simulink model "SimiSnake3"  (R2018b)
settings: Solver=VariableStepAuto  StartTime=0.0  StopTime=10.0  RelTol=1e-3  EnableMultiTasking=on
PreLoadFcn:
  | robotParameters;
undefined symbols (not defined in the file or in its folder): X, Y, Z
libraries: sm_lib x38, nesl_utility x25, simulink x6
settings Model: Creator=Jake  LastModifiedBy=Jake
settings DataIOCC: LimitDataPoints=on
settings OptimizationCC: LifeSpan=inf
settings DebuggingCC: AllowSymbolicDim=off  SFUnexpectedBacktrackingDiag=warning  SFNoUnconditionalDefaultTransitionDiag=warning  SFExecutionAtInitializationDiag=none
settings SFSimCC: SimUseLocalCustomCode=off
settings RTWCC: RTWUseLocalCustomCode=off
settings CodeAppCC: StateflowObjectComments=on
settings GRTTargetCC: TargetLangStandard=C89/C90 (ANSI)  GeneratePreprocessorConditionals=Disable all
settings ConfigComp: CovMetricSettings=dw  CovHtmlReporting=on  CovSaveCumulativeToWorkspaceVar=on  CovSaveSingleToWorkspaceVar=on  CovExternalEMLEnable=off  CovSFcnEnable=off
settings SimscapeCC: SimscapeNominalValues="[{\"value\":\"10\",\"unit\":\"V\"},{\"value\":\"1\",\"unit\":\"A\"},{\"value\":\"10\",\"unit\":\"N*m\"},{\"value\":\"10\",\"unit\":\"bar\"},{\"value\":\"100\",\"unit\":\"kJ/kg\"},{\"value\":\"1\",\"unit\":\"kW\"},{\"value\":\"300\",\"unit\":\"K\"},{\"value\":\"100\",\"unit\":\"cm^3/s\"},{\"value\":\"1\",\"unit\":\"kN\"},{\"value\":\"1\",\"unit\":\"g/cm^3\"},{\"value\":\"1\",\"unit\":\"l\"},{\"value\":\"1\",\"unit\":\"cm^2\"},{\"value\":\"60\",\"unit\":\"Hz\"}]"  SimscapeLogType=all  SimscapeLogDataHistory=10000
settings ConfigurationSet: Description=SimMechanics 2G

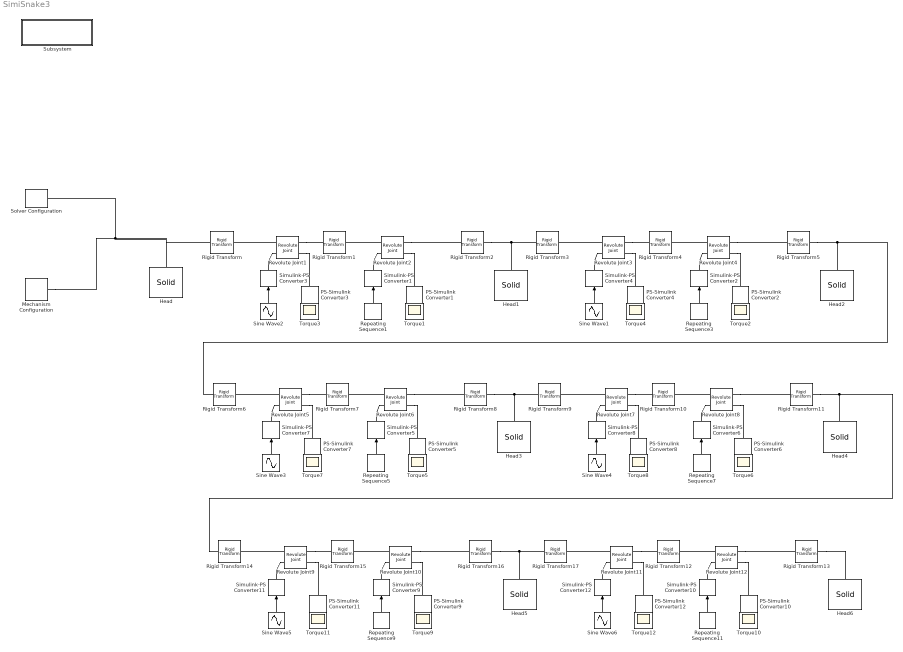
== system SimiSnake3 ==
  Head : sm_lib/Body Elements/Solid  InertiaType=CalculateFromGeometry  Mass=1  MassUnits=kg  CenterOfMass=[0 0 0]  CenterOfMassUnits=m  MomentsOfInertia=[1 1 1]  MomentsOfInertiaUnits=kg*m^2  ProductsOfInertia=[0 0 0]  ProductsOfInertiaUnits=kg*m^2  BasedOnType=Density  Density=0  DensityUnits=kg/m^3  DoExposeReferenceFrame=on  SerializedFrames=<Frames/>  GraphicType=FromGeometry  MarkerShape=Sphere  MarkerSize=10  GraphicVisPropType=SimpleVisualProperties  GraphicDiffuseColor=[1.0 0.0 0.2]  GraphicSpecularColor=[0.5 0.5 0.5 1.0]  GraphicAmbientColor=[0.15 0.15 0.15 1.0]  GraphicEmissiveColor=[0.0 0.0 0.0 1.0]  GraphicShininess=75  GraphicOpacity=1.0  GeometryShape=Cylinder  RectangleSize=[1 1]  RectangleSizeUnits=m  BrickDimensions=[1 1 1]  BrickDimensionUnits=m  CylinderRadius=1  CylinderRadiusUnits=cm  CylinderLength=10  CylinderLengthUnits=cm  SphereRadius=1  SphereRadiusUnits=m  EllipsoidRadii=[1 1 1]  EllipsoidRadiiUnits=m  ExtrusionCrossSection=[1 1; -1 1; -1 -1; 1 -1]  ExtrusionCrossSectionUnits=m  ExtrusionLength=1  ExtrusionLengthUnits=m  PolygonNumSides=3  PolygonOuterRadius=1  PolygonOuterRadiusUnits=m  ExtGeomFileType=STEP  ExtGeomFileUnits=m  RevolutionCrossSection=[1 1; 1 -1; 2 -1; 2 1]  RevolutionCrossSectionUnits=m  RevolutionExtent=Full  RevolutionAngle=180  RevolutionAngleUnits=deg
  Head{1..6} (6 alike) : sm_lib/Body Elements/Solid  InertiaType=CalculateFromGeometry  Mass=1  MassUnits=kg  CenterOfMass=[0 0 0]  CenterOfMassUnits=m  MomentsOfInertia=[1 1 1]  MomentsOfInertiaUnits=kg*m^2  ProductsOfInertia=[0 0 0]  ProductsOfInertiaUnits=kg*m^2  BasedOnType=Density  Density=500  DensityUnits=kg/m^3  DoExposeReferenceFrame=on  SerializedFrames=<Frames/>  GraphicType=FromGeometry  MarkerShape=Sphere  MarkerSize=10  GraphicVisPropType=SimpleVisualProperties  GraphicDiffuseColor=[1.0 1.0 0.2]  GraphicSpecularColor=[0.5 0.5 0.5 1.0]  GraphicAmbientColor=[0.15 0.15 0.15 1.0]  GraphicEmissiveColor=[0.0 0.0 0.0 1.0]  GraphicShininess=75  GraphicOpacity=1.0  GeometryShape=Cylinder  RectangleSize=[1 1]  RectangleSizeUnits=m  BrickDimensions=[1 1 1]  BrickDimensionUnits=m  CylinderRadius=1  CylinderRadiusUnits=cm  CylinderLength=10  CylinderLengthUnits=cm  SphereRadius=1  SphereRadiusUnits=m  EllipsoidRadii=[1 1 1]  EllipsoidRadiiUnits=m  ExtrusionCrossSection=[1 1; -1 1; -1 -1; 1 -1]  ExtrusionCrossSectionUnits=m  ExtrusionLength=1  ExtrusionLengthUnits=m  PolygonNumSides=3  PolygonOuterRadius=1  PolygonOuterRadiusUnits=m  ExtGeomFileType=STEP  ExtGeomFileUnits=m  RevolutionCrossSection=[1 1; 1 -1; 2 -1; 2 1]  RevolutionCrossSectionUnits=m  RevolutionExtent=Full  RevolutionAngle=180  RevolutionAngleUnits=deg
  Mechanism Configuration : sm_lib/Utilities/Mechanism Configuration  UniformGravity=Constant  GravityVector=[0 0 0]  GravityUnits=m/s^2  LinearizationDelta=0.001
  PS-Simulink Converter{1..12} (12 alike) : nesl_utility/PS-Simulink Converter  PhysicalDomain=network_engine_domain  SubClassName=ps_output  LeftPortType=input  RightPortType=output  PseudoPeriodic=off  Frequencies=[]  Unit=N*m  AffineConversion=off
  Repeating Sequence1 : simulink/Sources/Repeating Sequence  rep_seq_t=[0 1 2 3 4 5 6 7 8 9 10]  rep_seq_y=[0 -0 -20 -0 20 -0 -20 -0 20 -0 -20]
  Repeating Sequence{3,5,7,9,11} (5 alike) : simulink/Sources/Repeating Sequence  rep_seq_t=[0 1 2 3 4 5 6 7 8 9 10]  rep_seq_y=[0 -0 0 -0 0 -0 0 -0 0 -0 0]
  Revolute Joint{1..12} (12 alike) : sm_lib/Joints/Revolute Joint  SenseConstraintForce=off  SenseConstraintForceX=off  SenseConstraintForceY=off  SenseConstraintForceZ=off  SenseConstraintTorque=off  SenseConstraintTorqueX=off  SenseConstraintTorqueY=off  SenseConstraintTorqueZ=off  SenseTotalForce=off  SenseTotalForceX=off  SenseTotalForceY=off  SenseTotalForceZ=off  SenseTotalTorque=off  SenseTotalTorqueX=off  SenseTotalTorqueY=off  SenseTotalTorqueZ=off  CompositeWrenchDir=FollowerOnBase  CompositeWrenchFrame=BaseFrame  EquilibriumPosition=0  EquilibriumPositionUnits=deg  SpringStiffness=0  SpringStiffnessUnits=N*m/deg  DampingCoefficient=0  DampingCoefficientUnits=N*m/(deg/s)  TorqueActuationMode=ComputedTorque  MotionActuationMode=InputMotion  SensePosition=off  SenseVelocity=off  SenseAcceleration=off  SenseTorqueForce=on  PositionTargetSpecify=off  PositionTargetPriority=High  PositionTargetValue=30  PositionTargetValueUnits=deg  VelocityTargetSpecify=off  VelocityTargetPriority=High  VelocityTargetValue=0  VelocityTargetValueUnits=deg/s
  Rigid Transform{,3,6,9,14,17} (6 alike) : sm_lib/Frames and Transforms/Rigid Transform  TranslationMethod=StandardAxis  TranslationStandardOffset=5  TranslationLengthUnit=cm  TranslationStandardAxis=-Z  TranslationCartesianOffset=[0 0 0]  TranslationROffset=0  TranslationROffsetUnits=m  TranslationZOffset=0  TranslationZOffsetUnits=m  TranslationThetaOffset=0  TranslationThetaOffsetUnits=deg  RotationMethod=StandardAxis  RotationAngleUnits=deg  RotationStandardAxis=+X  RotationAngle=90  RotationArbitraryAxis=[0 0 1]  FollAlignAxisA=+X  BaseAlignAxisA=+Y  FollAlignAxisB=+Y  BaseAlignAxisB=+Z  RotationSequenceAxes=FollowerAxes  RotationSequence=XYX  RotationSequenceAngles=[0 0 0]  RotationSequenceAnglesUnits=deg  RotationMatrix=[1 0 0; 0 1 0; 0 0 1]
  Rigid Transform{1,4,7,10,12,15} (6 alike) : sm_lib/Frames and Transforms/Rigid Transform  TranslationMethod=None  TranslationStandardOffset=5  TranslationLengthUnit=cm  TranslationStandardAxis=-Z  TranslationCartesianOffset=[0 0 0]  TranslationROffset=0  TranslationROffsetUnits=m  TranslationZOffset=0  TranslationZOffsetUnits=m  TranslationThetaOffset=0  TranslationThetaOffsetUnits=deg  RotationMethod=StandardAxis  RotationAngleUnits=deg  RotationStandardAxis=+X  RotationAngle=90  RotationArbitraryAxis=[0 0 1]  FollAlignAxisA=+X  BaseAlignAxisA=+Y  FollAlignAxisB=+Y  BaseAlignAxisB=+Z  RotationSequenceAxes=FollowerAxes  RotationSequence=XYX  RotationSequenceAngles=[0 0 0]  RotationSequenceAnglesUnits=deg  RotationMatrix=[1 0 0; 0 1 0; 0 0 1]
  Rigid Transform{2,5,8,11,13,16} (6 alike) : sm_lib/Frames and Transforms/Rigid Transform  TranslationMethod=StandardAxis  TranslationStandardOffset=5  TranslationLengthUnit=cm  TranslationStandardAxis=+Z  TranslationCartesianOffset=[0 0 0]  TranslationROffset=0  TranslationROffsetUnits=m  TranslationZOffset=0  TranslationZOffsetUnits=m  TranslationThetaOffset=0  TranslationThetaOffsetUnits=deg  RotationMethod=StandardAxis  RotationAngleUnits=deg  RotationStandardAxis=-X  RotationAngle=180  RotationArbitraryAxis=[0 0 1]  FollAlignAxisA=+X  BaseAlignAxisA=+Y  FollAlignAxisB=+Y  BaseAlignAxisB=+Z  RotationSequenceAxes=FollowerAxes  RotationSequence=XYX  RotationSequenceAngles=[0 0 0]  RotationSequenceAnglesUnits=deg  RotationMatrix=[1 0 0; 0 1 0; 0 0 1]
  Simulink-PS Converter{1..12} (12 alike) : nesl_utility/Simulink-PS Converter  PhysicalDomain=network_engine_domain  SubClassName=ps_input  LeftPortType=input  RightPortType=output  PseudoPeriodic=off  Frequencies=[]  NoiseDistribution=none  NoiseParameters=[]  Unit=deg  AffineConversion=off  FilteringAndDerivatives=filter  SimscapeFilterOrder=2  InputFilterTimeConstant=.01  UdotUserProvided=1
  Sine Wave1 : Sin  Amplitude=80  Frequency=5  Phase=-pi/2  SampleTime=0
  Sine Wave2 : Sin  Amplitude=80  Frequency=5  SampleTime=0
  Sine Wave3 : Sin  Amplitude=80  Frequency=5  Phase=-pi*(2/2)  SampleTime=0
  Sine Wave4 : Sin  Amplitude=80  Frequency=5  Phase=-pi*(3/2)  SampleTime=0
  Sine Wave5 : Sin  Amplitude=80  Frequency=5  Phase=-pi*(4/2)  SampleTime=0
  Sine Wave6 : Sin  Amplitude=80  Frequency=5  Phase=-pi*(5/2)  SampleTime=0
  Solver Configuration : nesl_utility/Solver Configuration  PhysicalDomain=network_engine_domain  SubClassName=solver  LeftPortType=input  RightPortType=generic  Tones=[]  Harmonics=[]  SimulateNoise=off  Profile=off  UseLocalSampling=off  EnableSwitchedLinearOptims=on  FrequencyDomain=off  UseCCode=off  RelTol=0.001  AbsTol=1e-06  MinStep=1e-09  ToWorkspace=off  RevertToSquareIcSolve=off  NumHomotopyIterations=100  PhasorMode=off  PhasorModeNumHarmonics=1  DoDC=off  ResidualTolerance=1e-09  UseLocalSolver=off  LocalSolverChoice=NE_BACKWARD_EULER_ADVANCER  LocalSolverSampleTime=0.001  DoFixedCost=off  MaxNonlinIter=3  MaxModeIter=2  LinearAlgebra=Sparse  EquationFormulation=NE_TIME_EF  DelaysMemoryBudget=1024  AutomaticFiltering=on  FilteringTimeConstant=0.001  PartitionStorageMethod=AS_NEEDED  PartitionMemoryBudget=1024
  Subsystem : Subsystem
      settings: OpenFcn=open_system('sm_lib')
      mask Display: disp(sprintf('Open Simscape Multibody\nLibrary'));
  Torque{1..12} (12 alike) : Scope
  wires:
  Sine Wave2/1 -> Simulink-PS Converter3/1
  PS-Simulink Converter3/1 -> Torque3/1
  Repeating Sequence1/1 -> Simulink-PS Converter1/1
  PS-Simulink Converter1/1 -> Torque1/1
  Repeating Sequence3/1 -> Simulink-PS Converter2/1
  PS-Simulink Converter2/1 -> Torque2/1
  Sine Wave1/1 -> Simulink-PS Converter4/1
  PS-Simulink Converter4/1 -> Torque4/1
  Repeating Sequence5/1 -> Simulink-PS Converter5/1
  PS-Simulink Converter5/1 -> Torque5/1
  Sine Wave4/1 -> Simulink-PS Converter8/1
  PS-Simulink Converter6/1 -> Torque6/1
  Repeating Sequence7/1 -> Simulink-PS Converter6/1
  PS-Simulink Converter8/1 -> Torque8/1
  Sine Wave3/1 -> Simulink-PS Converter7/1
  PS-Simulink Converter7/1 -> Torque7/1
  PS-Simulink Converter9/1 -> Torque9/1
  Repeating Sequence9/1 -> Simulink-PS Converter9/1
  Sine Wave6/1 -> Simulink-PS Converter12/1
  Sine Wave5/1 -> Simulink-PS Converter11/1
  PS-Simulink Converter11/1 -> Torque11/1
  Repeating Sequence11/1 -> Simulink-PS Converter10/1
  PS-Simulink Converter12/1 -> Torque12/1
  PS-Simulink Converter10/1 -> Torque10/1
  connections:
  Mechanism Configuration/RConn1 -- Rigid Transform/LConn1 -- Head/RConn1 -- Solver Configuration/RConn1
  Revolute Joint1/RConn2 -- PS-Simulink Converter3/LConn1
  Simulink-PS Converter3/RConn1 -- Revolute Joint1/LConn2
  Revolute Joint1/RConn1 -- Rigid Transform1/LConn1
  Revolute Joint1/LConn1 -- Rigid Transform/RConn1
  Rigid Transform2/RConn1 -- Rigid Transform3/LConn1 -- Head1/RConn1
  Revolute Joint2/LConn1 -- Rigid Transform1/RConn1
  Revolute Joint2/RConn1 -- Rigid Transform2/LConn1
  Revolute Joint2/RConn2 -- PS-Simulink Converter1/LConn1
  Simulink-PS Converter1/RConn1 -- Revolute Joint2/LConn2
  Revolute Joint3/RConn2 -- PS-Simulink Converter4/LConn1
  Revolute Joint4/RConn2 -- PS-Simulink Converter2/LConn1
  Revolute Joint3/RConn1 -- Rigid Transform4/LConn1
  Rigid Transform5/RConn1 -- Rigid Transform6/LConn1 -- Head2/RConn1
  Revolute Joint4/LConn1 -- Rigid Transform4/RConn1
  Revolute Joint3/LConn1 -- Rigid Transform3/RConn1
  Simulink-PS Converter4/RConn1 -- Revolute Joint3/LConn2
  Simulink-PS Converter2/RConn1 -- Revolute Joint4/LConn2
  Revolute Joint4/RConn1 -- Rigid Transform5/LConn1
  Rigid Transform8/RConn1 -- Rigid Transform9/LConn1 -- Head3/RConn1
  Revolute Joint8/RConn1 -- Rigid Transform11/LConn1
  Revolute Joint6/LConn1 -- Rigid Transform7/RConn1
  Revolute Joint6/RConn1 -- Rigid Transform8/LConn1
  Revolute Joint5/RConn2 -- PS-Simulink Converter7/LConn1
  Simulink-PS Converter6/RConn1 -- Revolute Joint8/LConn2
  Revolute Joint6/RConn2 -- PS-Simulink Converter5/LConn1
  Simulink-PS Converter5/RConn1 -- Revolute Joint6/LConn2
  Rigid Transform11/RConn1 -- Rigid Transform14/LConn1 -- Head4/RConn1
  Revolute Joint7/LConn1 -- Rigid Transform9/RConn1
  Simulink-PS Converter8/RConn1 -- Revolute Joint7/LConn2
  Revolute Joint8/RConn2 -- PS-Simulink Converter6/LConn1
  Simulink-PS Converter7/RConn1 -- Revolute Joint5/LConn2
  Revolute Joint7/RConn2 -- PS-Simulink Converter8/LConn1
  Revolute Joint8/LConn1 -- Rigid Transform10/RConn1
  Revolute Joint5/LConn1 -- Rigid Transform6/RConn1
  Revolute Joint5/RConn1 -- Rigid Transform7/LConn1
  Revolute Joint7/RConn1 -- Rigid Transform10/LConn1
  Rigid Transform16/RConn1 -- Rigid Transform17/LConn1 -- Head5/RConn1
  Simulink-PS Converter11/RConn1 -- Revolute Joint9/LConn2
  Revolute Joint9/LConn1 -- Rigid Transform14/RConn1
  Rigid Transform13/RConn1 -- Head6/RConn1
  Simulink-PS Converter12/RConn1 -- Revolute Joint11/LConn2
  Revolute Joint10/LConn1 -- Rigid Transform15/RConn1
  Revolute Joint9/RConn1 -- Rigid Transform15/LConn1
  Revolute Joint11/RConn2 -- PS-Simulink Converter12/LConn1
  Simulink-PS Converter9/RConn1 -- Revolute Joint10/LConn2
  Revolute Joint12/LConn1 -- Rigid Transform12/RConn1
  Simulink-PS Converter10/RConn1 -- Revolute Joint12/LConn2
  Revolute Joint10/RConn1 -- Rigid Transform16/LConn1
  Revolute Joint11/RConn1 -- Rigid Transform12/LConn1
  Revolute Joint11/LConn1 -- Rigid Transform17/RConn1
  Revolute Joint12/RConn1 -- Rigid Transform13/LConn1
  Revolute Joint12/RConn2 -- PS-Simulink Converter10/LConn1
  Revolute Joint10/RConn2 -- PS-Simulink Converter9/LConn1
  Revolute Joint9/RConn2 -- PS-Simulink Converter11/LConn1

== system SimiSnake3/Subsystem ==
